simulink subsystem "subsystem_slip_modulation_simplified"  (R2022a)
settings: Solver=VariableStepAuto  StartTime=0.0  StopTime=10.0  RelTol=1e-3
libraries: neuromorphic_blocks x11
settings Model: Creator=chris  LastModifiedBy=chris

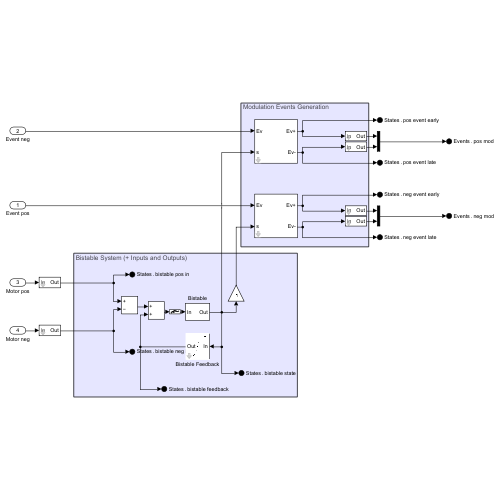
[thumbnail: Simulink's stored preview of the top-level diagram]
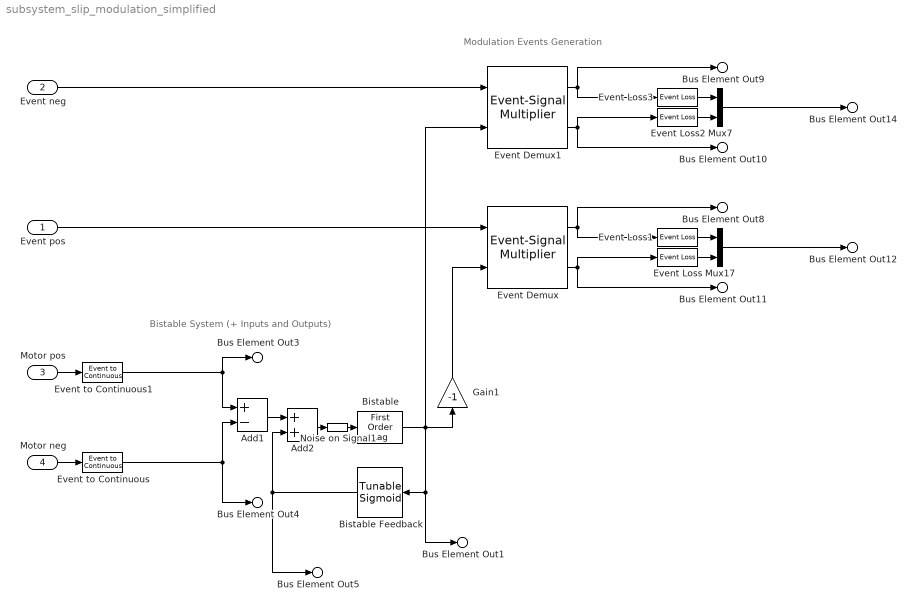
== system subsystem_slip_modulation_simplified ==
  note: Bistable System (+ Inputs and Outputs)
  note: Modulation Events Generation
  Event pos : Inport
  Event neg : Inport  Port=2
  Motor pos : Inport  Port=3
  Motor neg : Inport  Port=4
  Add1 : Sum  Inputs=+-
  Add2 : Sum
  Bistable : neuromorphic_blocks/First Order Lag  gain=1  timescale=timescale  rel_timescale=0.1
      settings: SourceProductName=Neuromorphic Toolbox
  Bistable Feedback : neuromorphic_blocks/Tunable Sigmoid  nonlinearity_type=Tanh  gain_source=Internal  gain=5  bias=0  slope=1
      settings: SourceProductName=Neuromorphic Toolbox
  Event Demux : neuromorphic_blocks/Auxiliary Blocks/Event-Signal Multiplier  symmetric_box=off  dsyn_signal_pos=0  dsyn_signal_neg=0  dsyn_signal_neg_save=0  gain_signal_pos=1  gain_signal_neg=1  gain_signal_neg_save=1  input=Events  gsyn_pos=20  gsyn_neg=20  gsyn_neg_save=20  dsyn_event_pos=10  dsyn_event_neg=10  dsyn_event_neg_save=10  gain_event_pos=20  gain_event_neg=20  gain_event_neg_save=20
      settings: SourceProductName=NeurCont Toolbox
  Event Demux1 : neuromorphic_blocks/Auxiliary Blocks/Event-Signal Multiplier  symmetric_box=off  dsyn_signal_pos=0  dsyn_signal_neg=0  dsyn_signal_neg_save=0  gain_signal_pos=1  gain_signal_neg=1  gain_signal_neg_save=1  input=Events  gsyn_pos=20  gsyn_neg=20  gsyn_neg_save=20  dsyn_event_pos=10  dsyn_event_neg=10  dsyn_event_neg_save=10  gain_event_pos=20  gain_event_neg=20  gain_event_neg_save=20
      settings: SourceProductName=NeurCont Toolbox
  Event Loss{,1..3} (4 alike) : neuromorphic_blocks/Events Transmission Blocks/Event Loss  loss_prob=prob_event_loss  seed=-1  seed_mem=randi([0, 100000])
      settings: SourceProductName=Neuromorphic Toolbox
  Event to Continuous : neuromorphic_blocks/Events Transmission Blocks/Event to Continuous  gain=20
      settings: SourceProductName=Neuromorphic Toolbox
  Event to Continuous1 : neuromorphic_blocks/Events Transmission Blocks/Event to Continuous  gain=20
      settings: SourceProductName=Neuromorphic Toolbox
  Gain1 : Gain  Gain=-1
  Mux17 : Mux  Inputs=2
  Mux7 : Mux  Inputs=2
  Noise on Signal1 : neuromorphic_blocks/Auxiliary Blocks/Noise on Signal  noise_pwr=noisePwr  timescale=timescale  rel_timescale=rel_noise  seed=-1  seed_mem=randi([0, 100000])
      settings: SourceProductName=NeurCont Toolbox
  Bus Element Out14 : Outport  PortName=Events  Element=pos mod
  Bus Element Out12 : Outport  PortName=Events  Element=neg mod
  Bus Element Out9 : Outport  Port=2  PortName=States  Element=pos event early
  Bus Element Out10 : Outport  Port=2  PortName=States  Element=pos event late
  Bus Element Out8 : Outport  Port=2  PortName=States  Element=neg event early
  Bus Element Out11 : Outport  Port=2  PortName=States  Element=neg event late
  Bus Element Out1 : Outport  Port=2  PortName=States  Element=bistable state
  Bus Element Out3 : Outport  Port=2  PortName=States  Element=bistable pos in
  Bus Element Out4 : Outport  Port=2  PortName=States  Element=bistable neg in
  Bus Element Out5 : Outport  Port=2  PortName=States  Element=bistable feedback
  wires:
  Bistable/1 -> Bistable Feedback/1, Bus Element Out1/1, Gain1/1, Event Demux1/2
  Event to Continuous1/1 -> Add1/1, Bus Element Out3/1
  Event to Continuous/1 -> Add1/2, Bus Element Out4/1
  Add1/1 -> Add2/1
  Motor pos/1 -> Event to Continuous1/1
  Motor neg/1 -> Event to Continuous/1
  Gain1/1 -> Event Demux/2
  Mux7/1 -> Bus Element Out14/1
  Mux17/1 -> Bus Element Out12/1
  Event Demux/1 -> Bus Element Out8/1, Event Loss1/1
  Event Demux/2 -> Bus Element Out11/1, Event Loss/1
  Event Loss/1 -> Mux17/2
  Event Loss1/1 -> Mux17/1
  Event Demux1/1 -> Bus Element Out9/1, Event Loss3/1
  Event Demux1/2 -> Bus Element Out10/1, Event Loss2/1
  Event Loss2/1 -> Mux7/2
  Event Loss3/1 -> Mux7/1
  Bistable Feedback/1 -> Add2/2, Bus Element Out5/1
  Add2/1 -> Noise on Signal1/1
  Noise on Signal1/1 -> Bistable/1
  Event pos/1 -> Event Demux/1
  Event neg/1 -> Event Demux1/1
